simulink model "px4TestBasic"  (R2025b)
settings: Solver=FixedStepDiscrete  StartTime=0.0  StopTime=10.0  FixedStep=1/200  RelTol=1e-3
undefined symbols (not defined in the file or in its folder): position, timestamp
libraries: px4_lib x20
settings Model: Creator=jack  LastModifiedBy=jack
settings OptimizationCC: DefaultParameterBehavior=Inlined  DefaultUnderspecifiedDataType=single  EnhancedBackFolding=on  CachingGlobalReferences=on  StrengthReduction=on  PassReuseOutputArgsAs=Individual arguments  StateBitsets=on  DataBitsets=on  MaxStackSize=64  OptimizeBlockOrder=speed  DifferentSizesBufferReuse=on  EfficientTunableParamExpr=on
settings DebuggingCC: ParameterPrecisionLossMsg=none  ParameterTunabilityLossMsg=error  UnnecessaryDatatypeConvMsg=warning  UnconnectedInputMsg=warning  UnconnectedOutputMsg=warning  UnconnectedLineMsg=warning
settings HardwareCC: ProdBitPerPointer=32.0  ProdBitPerSizeT=32.0  ProdBitPerPtrDiffT=32.0  ProdLargestAtomicInteger=Long  ProdLargestAtomicFloat=Double  ProdWordSize=32.0  ProdLongLongMode=on  ProdHWDeviceType=ARM Compatible->ARM Cortex-M
settings SFSimCC: SimCustomHeaderCode="#include \"px4_simulink_api.h\""  SimUserSources=px4_simulink_api.c  MATLABDynamicMemAlloc=off
settings RTWCC: SystemTargetFile=ert.tlc  GenCodeOnly=on  TemplateMakefile=ert_default_tmf  PostCodeGenCommand=px4io.px4API.runPostCodeGen(buildInfo)  CustomHeaderCode="#include \"px4_simulink_api.h\""  BuildConfiguration=Faster Runs  DataTypeReplacement=CDataTypesFixedWidth  Description=Embedded Coder
settings CodeAppCC: ForceParamTrailComments=on  IgnoreCustomStorageClasses=off  OperatorAnnotations=on  SimulinkDataObjDesc=on  SFDataObjDesc=on  InsertBlockDesc=on
settings ERTTargetCC: ExtModeTransport=2.0  ExtModeStaticAlloc=on  ExtModeMexFile=ext_xcp  ExtModeIntrfLevel=Level2 - Open  InlinedParameterPlacement=Hierarchical  RootIOFormat=Structure reference  ERTCustomFileTemplate=example_file_process.tlc  MaxIdInt64=INT64_MAX  MinIdInt64=INT64_MIN  MaxIdUint64=UINT64_MAX  MaxIdInt32=INT32_MAX  MinIdInt32=INT32_MIN  MaxIdUint32=UINT32_MAX  MaxIdInt16=INT16_MAX  MinIdInt16=INT16_MIN  MaxIdUint16=UINT16_MAX  MaxIdInt8=INT8_MAX  MinIdInt8=INT8_MIN  MaxIdUint8=UINT8_MAX  SupportVariableSizeSignals=on  ParenthesesLevel=Standards  CastingMode=Standards

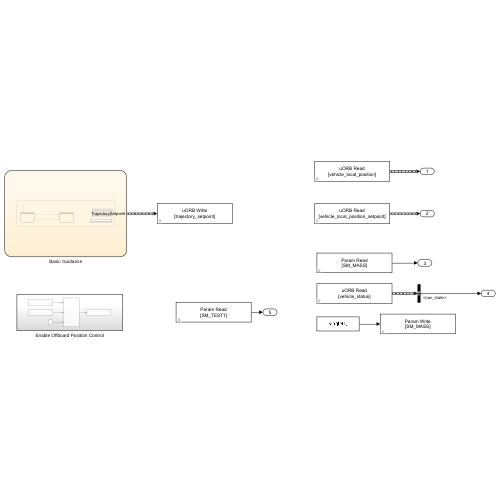
[thumbnail: Simulink's stored preview of the top-level diagram]
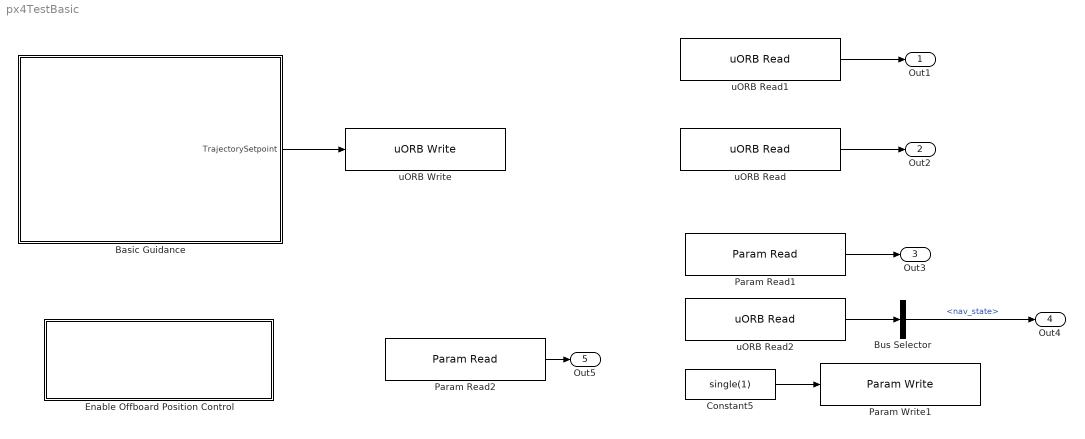
== system px4TestBasic ==
  Basic Guidance : Stateflow chart  TreatAsAtomicUnit=on
  Bus Selector : BusSelector  OutputSignals=nav_state
  Constant5 : Constant  Value=single(1)
  Enable Offboard Position Control : Subsystem
  Param Read1 : px4_lib/Param Read  param_name=SM_MASS  param_type=single  sample_time=-1
  Param Read2 : px4_lib/Param Read  param_name=SM_TEST1  param_type=single  sample_time=-1
  Param Write1 : px4_lib/Param Write  param_name=SM_MASS  param_type=single  sample_time=-1
  uORB Read : px4_lib/uORB Read  uorb_topic=vehicle_local_position_setpoint  uorb_variant=vehicle_local_position_setpoint  sample_time=1/200
  uORB Read1 : px4_lib/uORB Read  uorb_topic=vehicle_local_position  uorb_variant=vehicle_local_position  sample_time=1/200
  uORB Read2 : px4_lib/uORB Read  uorb_topic=vehicle_status  uorb_variant=vehicle_status  sample_time=1/200
  uORB Write : px4_lib/uORB Write  uorb_topic=trajectory_setpoint  uorb_variant=trajectory_setpoint  sample_time=1/200
  Out1 : Outport
  Out2 : Outport  Port=2
  Out3 : Outport  Port=3
  Out4 : Outport  Port=4
  Out5 : Outport  Port=5
  wires:
  uORB Read1/1 -> Out1/1
  uORB Read/1 -> Out2/1
  Param Read1/1 -> Out3/1
  Constant5/1 -> Param Write1/1
  Basic Guidance/1(TrajectorySetpoint) -> uORB Write/1
  uORB Read2/1 -> Bus Selector/1
  Bus Selector/1 -> Out4/1  "<nav_state>"
  Param Read2/1 -> Out5/1

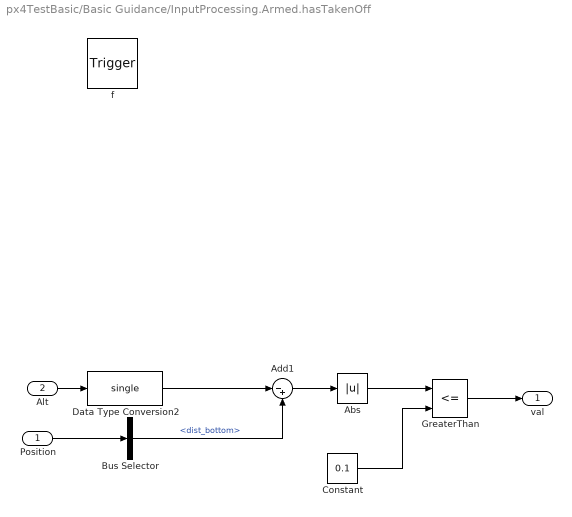
== system px4TestBasic/Basic Guidance/InputProcessing.Armed.hasTakenOff ==
  Position : Inport  OutDataTypeStr=Bus: vehicle_local_position_s  PortDimensions=1
  Alt : Inport  Port=2  OutDataTypeStr=double  PortDimensions=1
  f : TriggerPort  TriggerType=function-call  VariantControl=(inherit)
      settings: CopyFcn=Stateflow.SLINSF.SimulinkMan.removeBlockPreDeleteFcn  PreDeleteFcn=Stateflow.SLINSF.SimulinkMan.unsafePredeleteFcn
  Abs : Abs  SaturateOnIntegerOverflow=off
  Add1 : Sum  Inputs=|-+
  Bus Selector : BusSelector  OutputSignals=dist_bottom
  Constant : Constant  Value=0.1
  Data Type Conversion2 : DataTypeConversion  OutDataTypeStr=single  SaturateOnIntegerOverflow=off  RndMeth=Floor
  GreaterThan : RelationalOperator  Operator=<=  OutDataTypeStr=boolean  RndMeth=Simplest  InputSameDT=off
  val : Outport  PortDimensions=1
  wires:
  Bus Selector/1 -> Add1/2  "<dist_bottom>"
  GreaterThan/1 -> val/1
  Position/1 -> Bus Selector/1
  Alt/1 -> Data Type Conversion2/1
  Data Type Conversion2/1 -> Add1/1
  Add1/1 -> Abs/1
  Constant/1 -> GreaterThan/2
  Abs/1 -> GreaterThan/1

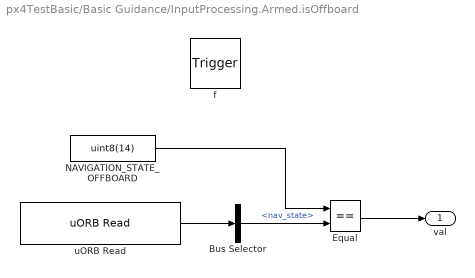
== system px4TestBasic/Basic Guidance/InputProcessing.Armed.isOffboard ==
  f : TriggerPort  TriggerType=function-call  VariantControl=(inherit)
      settings: CopyFcn=Stateflow.SLINSF.SimulinkMan.removeBlockPreDeleteFcn  PreDeleteFcn=Stateflow.SLINSF.SimulinkMan.unsafePredeleteFcn
  Bus Selector : BusSelector  OutputSignals=nav_state
  Equal : RelationalOperator  Operator===  OutDataTypeStr=boolean  RndMeth=Simplest  InputSameDT=off
  NAVIGATION_STATE_OFFBOARD : Constant  Value=uint8(14)
  uORB Read : px4_lib/uORB Read  uorb_topic=vehicle_status  uorb_variant=vehicle_status  sample_time=-1
  val : Outport
  wires:
  uORB Read/1 -> Bus Selector/1
  NAVIGATION_STATE_OFFBOARD/1 -> Equal/1
  Bus Selector/1 -> Equal/2  "<nav_state>"
  Equal/1 -> val/1

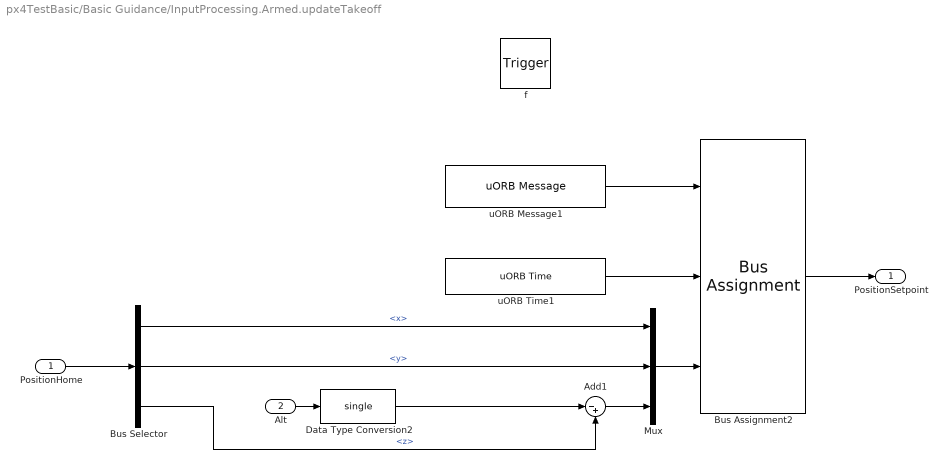
== system px4TestBasic/Basic Guidance/InputProcessing.Armed.updateTakeoff ==
  PositionHome : Inport  OutDataTypeStr=Bus: vehicle_local_position_s  PortDimensions=1
  Alt : Inport  Port=2  OutDataTypeStr=double  PortDimensions=1
  f : TriggerPort  TriggerType=function-call  VariantControl=(inherit)
      settings: CopyFcn=Stateflow.SLINSF.SimulinkMan.removeBlockPreDeleteFcn  PreDeleteFcn=Stateflow.SLINSF.SimulinkMan.unsafePredeleteFcn
  Add1 : Sum  Inputs=|-+
  Bus Assignment2 : BusAssignment  AssignedSignals=timestamp,position
  Bus Selector : BusSelector  OutputSignals=x,y,z
  Data Type Conversion2 : DataTypeConversion  OutDataTypeStr=single  SaturateOnIntegerOverflow=off  RndMeth=Floor
  Mux : Mux  Inputs=3
  uORB Message1 : px4_lib/uORB Message  uorb_topic=trajectory_setpoint  uorb_variant=trajectory_setpoint  init_value=NaN  sample_time=-1
  uORB Time1 : px4_lib/uORB Time  sample_time=-1
  PositionSetpoint : Outport  OutDataTypeStr=Bus: trajectory_setpoint_s  PortDimensions=1
  wires:
  uORB Message1/1 -> Bus Assignment2/1
  uORB Time1/1 -> Bus Assignment2/2
  Bus Selector/3 -> Add1/2  "<z>"
  Bus Assignment2/1 -> PositionSetpoint/1
  PositionHome/1 -> Bus Selector/1
  Alt/1 -> Data Type Conversion2/1
  Data Type Conversion2/1 -> Add1/1
  Add1/1 -> Mux/3
  Bus Selector/2 -> Mux/2  "<y>"
  Bus Selector/1 -> Mux/1  "<x>"
  Mux/1 -> Bus Assignment2/3

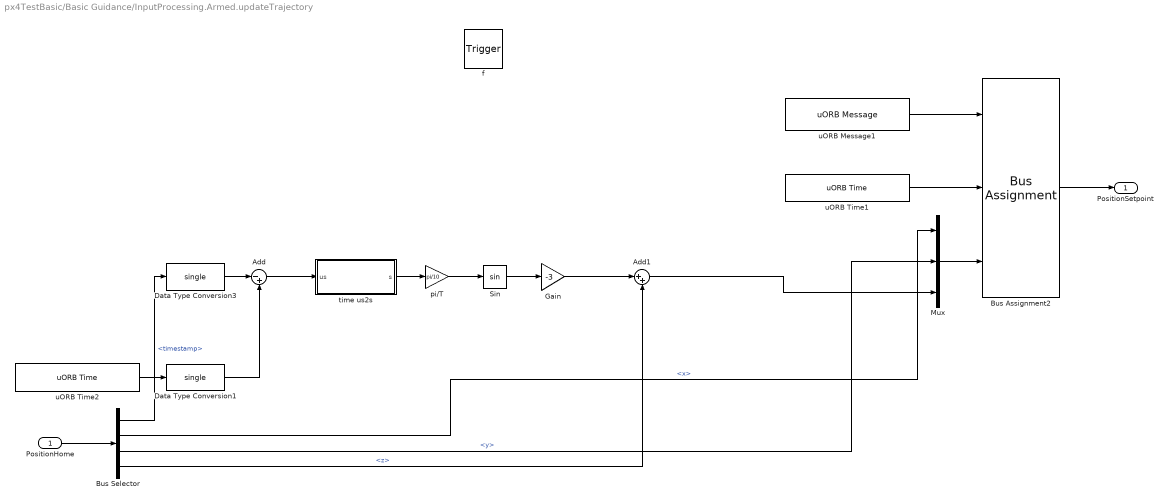
== system px4TestBasic/Basic Guidance/InputProcessing.Armed.updateTrajectory ==
  PositionHome : Inport  OutDataTypeStr=Bus: vehicle_local_position_s  PortDimensions=1
  f : TriggerPort  TriggerType=function-call  VariantControl=(inherit)
      settings: CopyFcn=Stateflow.SLINSF.SimulinkMan.removeBlockPreDeleteFcn  PreDeleteFcn=Stateflow.SLINSF.SimulinkMan.unsafePredeleteFcn
  Add : Sum  Inputs=|-+
  Add1 : Sum  Inputs=|++
  Bus Assignment2 : BusAssignment  AssignedSignals=timestamp,position
  Bus Selector : BusSelector  OutputSignals=timestamp,x,y,z
  Data Type Conversion1 : DataTypeConversion  OutDataTypeStr=single  SaturateOnIntegerOverflow=off  RndMeth=Floor
  Data Type Conversion3 : DataTypeConversion  OutDataTypeStr=single  SaturateOnIntegerOverflow=off  RndMeth=Floor
  Gain : Gain  Gain=-3  ParamDataTypeStr=single
  Mux : Mux  Inputs=3
  Sin : Trigonometry  OutputSignalType=real
  pi/T : Gain  Gain=pi/10  ParamDataTypeStr=single
  time us2s : Subsystem
  uORB Message1 : px4_lib/uORB Message  uorb_topic=trajectory_setpoint  uorb_variant=trajectory_setpoint  init_value=NaN  sample_time=-1
  uORB Time1 : px4_lib/uORB Time  sample_time=-1
  uORB Time2 : px4_lib/uORB Time  sample_time=-1
  PositionSetpoint : Outport  OutDataTypeStr=Bus: trajectory_setpoint_s  PortDimensions=1
  wires:
  uORB Time2/1 -> Data Type Conversion1/1
  uORB Message1/1 -> Bus Assignment2/1
  Bus Selector/1 -> Data Type Conversion3/1  "<timestamp>"
  pi/T/1 -> Sin/1
  uORB Time1/1 -> Bus Assignment2/2
  Add/1 -> time us2s/1(us)
  time us2s/1(s) -> pi/T/1
  Sin/1 -> Gain/1
  Bus Selector/4 -> Add1/2  "<z>"
  Bus Assignment2/1 -> PositionSetpoint/1
  PositionHome/1 -> Bus Selector/1
  Data Type Conversion1/1 -> Add/2
  Data Type Conversion3/1 -> Add/1
  Gain/1 -> Add1/1
  Bus Selector/2 -> Mux/1  "<x>"
  Bus Selector/3 -> Mux/2  "<y>"
  Add1/1 -> Mux/3
  Mux/1 -> Bus Assignment2/3

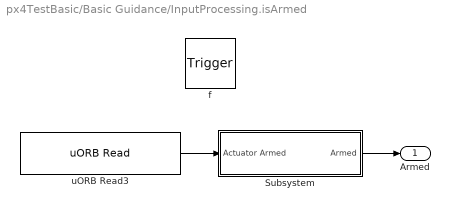
== system px4TestBasic/Basic Guidance/InputProcessing.isArmed ==
  f : TriggerPort  TriggerType=function-call  VariantControl=(inherit)
      settings: CopyFcn=Stateflow.SLINSF.SimulinkMan.removeBlockPreDeleteFcn  PreDeleteFcn=Stateflow.SLINSF.SimulinkMan.unsafePredeleteFcn
  Subsystem : Subsystem
  uORB Read3 : px4_lib/uORB Read  uorb_topic=actuator_armed  uorb_variant=actuator_armed  sample_time=-1
  Armed : Outport
  wires:
  uORB Read3/1 -> Subsystem/1(Actuator Armed)
  Subsystem/1(Armed) -> Armed/1

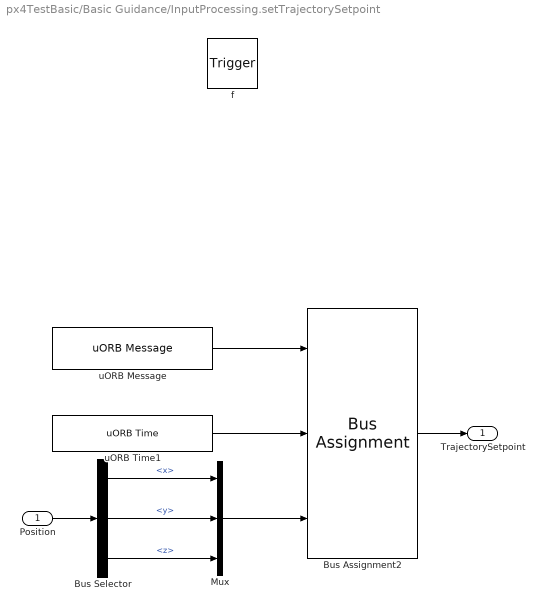
== system px4TestBasic/Basic Guidance/InputProcessing.setTrajectorySetpoint ==
  Position : Inport  OutDataTypeStr=Bus: vehicle_local_position_s  PortDimensions=1
  f : TriggerPort  TriggerType=function-call  VariantControl=(inherit)
      settings: CopyFcn=Stateflow.SLINSF.SimulinkMan.removeBlockPreDeleteFcn  PreDeleteFcn=Stateflow.SLINSF.SimulinkMan.unsafePredeleteFcn
  Bus Assignment2 : BusAssignment  AssignedSignals=timestamp,position
  Bus Selector : BusSelector  OutputSignals=x,y,z
  Mux : Mux  Inputs=3
  uORB Message : px4_lib/uORB Message  uorb_topic=trajectory_setpoint  uorb_variant=trajectory_setpoint  init_value=NaN  sample_time=-1
  uORB Time1 : px4_lib/uORB Time  sample_time=-1
  TrajectorySetpoint : Outport  OutDataTypeStr=Bus: trajectory_setpoint_s  PortDimensions=1
  wires:
  uORB Message/1 -> Bus Assignment2/1
  Bus Assignment2/1 -> TrajectorySetpoint/1
  uORB Time1/1 -> Bus Assignment2/2
  Position/1 -> Bus Selector/1
  Bus Selector/3 -> Mux/3  "<z>"
  Bus Selector/2 -> Mux/2  "<y>"
  Bus Selector/1 -> Mux/1  "<x>"
  Mux/1 -> Bus Assignment2/3

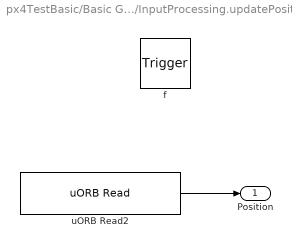
== system px4TestBasic/Basic Guidance/InputProcessing.updatePosition ==
  f : TriggerPort  TriggerType=function-call  VariantControl=(inherit)
      settings: CopyFcn=Stateflow.SLINSF.SimulinkMan.removeBlockPreDeleteFcn  PreDeleteFcn=Stateflow.SLINSF.SimulinkMan.unsafePredeleteFcn
  uORB Read2 : px4_lib/uORB Read  uorb_topic=vehicle_local_position  uorb_variant=vehicle_local_position  sample_time=-1
  Position : Outport
  wires:
  uORB Read2/1 -> Position/1

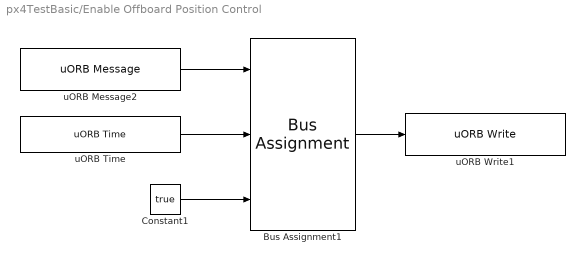
== system px4TestBasic/Enable Offboard Position Control ==
  Bus Assignment1 : BusAssignment  AssignedSignals=timestamp,position
  Constant1 : Constant  Value=true
  uORB Message2 : px4_lib/uORB Message  uorb_topic=offboard_control_mode  uorb_variant=offboard_control_mode  init_value=0  sample_time=-1
  uORB Time : px4_lib/uORB Time  sample_time=-1
  uORB Write1 : px4_lib/uORB Write  uorb_topic=offboard_control_mode  uorb_variant=offboard_control_mode  sample_time=1/200
  wires:
  Constant1/1 -> Bus Assignment1/3
  Bus Assignment1/1 -> uORB Write1/1
  uORB Message2/1 -> Bus Assignment1/1
  uORB Time/1 -> Bus Assignment1/2

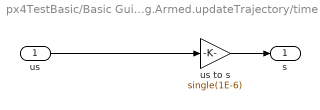
== system px4TestBasic/Basic Guidance/InputProcessing.Armed.updateTrajectory/time us2s ==
  us : Inport
  us to s : Gain  Gain=single(1E-6)  ParamDataTypeStr=single
  s : Outport
  wires:
  us/1 -> us to s/1
  us to s/1 -> s/1

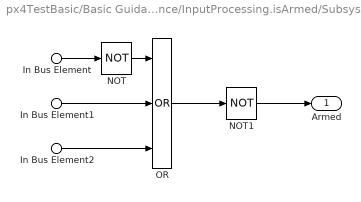
== system px4TestBasic/Basic Guidance/InputProcessing.isArmed/Subsystem ==
  In Bus Element : Inport  PortName=Actuator Armed  Element=armed
  In Bus Element1 : Inport  PortName=Actuator Armed  Element=lockdown
  In Bus Element2 : Inport  PortName=Actuator Armed  Element=in_esc_calibration_mode
  NOT : Logic  Operator=NOT  IconShape=distinctive  AllPortsSameDT=off  OutDataTypeStr=boolean
  NOT1 : Logic  Operator=NOT  IconShape=distinctive  AllPortsSameDT=off  OutDataTypeStr=boolean
  OR : Logic  Operator=OR  Inputs=3  IconShape=distinctive  AllPortsSameDT=off  OutDataTypeStr=boolean
  Armed : Outport
  wires:
  NOT1/1 -> Armed/1
  In Bus Element/1 -> NOT/1
  In Bus Element1/1 -> OR/2
  In Bus Element2/1 -> OR/3
  NOT/1 -> OR/1
  OR/1 -> NOT1/1

== stateflow chart px4TestBasic/Basic Guidance ==
  settings: updateMethod=DISCRETE  sampleTime=1/200
  state InputProcessing
    state Armed = isArmed [function]
    state Disarmed
      (default) -> (junction 60) : {
          | TrajectorySetpoint = setTrajectorySetpoint(PositionHome);
          | }
    state Armed
      state Takeoff
        entry:
        entry, during:
        TrajectorySetpoint = updateTakeoff(PositionHome, takeoff_altitude);
      state Flying
        entry:
        PositionTakenoff = updatePosition();
        entry, during:
        TrajectorySetpoint = updateTrajectory(PositionTakenoff);
      state Landed
        entry:
        takeoff_altitude = 10;
        PositionHome = updatePosition();
        entry, during:
        TrajectorySetpoint = setTrajectorySetpoint(PositionHome);
      state val = isOffboard [function]
      state PositionSetpoint = updateTrajectory(PositionHome) [function]
      state val = hasTakenOff(Position,Alt) [function]
      state PositionSetpoint = updateTakeoff(PositionHome, Alt) [function]
      (default) -> Landed
      Takeoff -> Flying [order 2] : [hasTakenOff(updatePosition(), takeoff_altitude)]
      Landed -> Takeoff : [isOffboard()]
      (junction 88) -> Landed : {PositionHome = updatePosition();}
      Takeoff -> (junction 83) [order 1] : [~isOffboard()]
      Flying -> (junction 84) : [~isOffboard()]
      (junction 83) -> (junction 88)
      (junction 84) -> (junction 83)
    state Position = updatePosition [function]
    state TrajectorySetpoint = setTrajectorySetpoint(Position) [function]
    (default) -> Disarmed : {
        | PositionHome = updatePosition();
        | TrajectorySetpoint = setTrajectorySetpoint(PositionHome);
        | }
    Disarmed -> Armed : [isArmed()]
    Armed -> Disarmed : [~isArmed()]
  data: Armed function_output; val function_output; PositionHome function_input Bus: vehicle_local_position_s size=1; PositionSetpoint function_output Bus: trajectory_setpoint_s size=1; Position function_input Bus: vehicle_local_position_s size=1; val function_output size=1; Alt function_input double size=1; PositionHome function_input Bus: vehicle_local_position_s size=1; PositionSetpoint function_output Bus: trajectory_setpoint_s size=1; Alt function_input double size=1; Position function_output; TrajectorySetpoint function_output Bus: trajectory_setpoint_s size=1; Position function_input Bus: vehicle_local_position_s size=1; PositionHome local Bus: vehicle_local_position_s size=1; TrajectorySetpoint output Bus: trajectory_setpoint_s size=1; takeoff_altitude local; PositionTakenoff local Bus: vehicle_local_position_s size=1
